simulink model "FourCellImplementation"  (R2020a)
settings: Solver=VariableStepAuto  StartTime=0.0  StopTime=10.0  RelTol=1e-3
libraries: powerlib x18
settings Model: Creator=HP  LastModifiedBy=HP

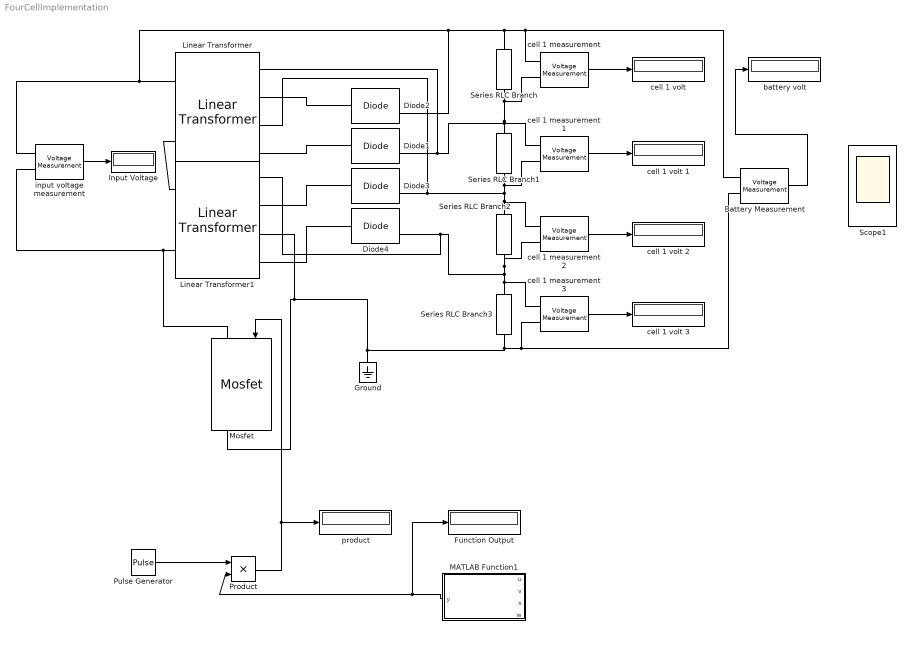
== system FourCellImplementation ==
  "Battery Measurement " : powerlib/Measurements/Voltage Measurement  PhasorSimulation=off  OutputType=Complex  PSBequivalent=0
  Diode{1..4} (4 alike) : powerlib/Power Electronics/Diode  Ron=0.001  Lon=0  Vf=0.8  IC=0  UseSnubber=0  Rs=500  Cs=250e-9  Measurements=on
  Function Output : Display
  Ground : powerlib/Elements/Ground  LConnTagsString=a
  Input Voltage : Display
  Linear Transformer : powerlib/Elements/Linear Transformer  UNITS=SI  NominalPower=[100 55000]  winding1=[10 0.02 45e-6]  winding2=[5 0.02 288e-6]  ThreeWindings=on  winding3=[5 0.02 288e-6]  RmLm=[1.0805e+06 2866]  Measurements=None  DataType=on
  Linear Transformer1 : powerlib/Elements/Linear Transformer  UNITS=SI  NominalPower=[100 55000]  winding1=[10 0.02 45e-6]  winding2=[5 0.02 288e-6]  ThreeWindings=on  winding3=[5 0.02 288e-6]  RmLm=[1.0805e+06 2866]  Measurements=None  DataType=on
  MATLAB Function1 : MATLAB Function  TreatAsAtomicUnit=on
  Mosfet : powerlib/Power Electronics/Mosfet  Ron=1.5  Lon=0  Rd=2  Vfd=0  IC=0  Rs=1500  Cs=288e-7  Measurements=on
  Product : Product
  Pulse Generator : DiscretePulseGenerator  PulseType=Time based  Period=10  PulseWidth=50
  Scope1 : Scope  NumInputPorts=5
  Series RLC Branch : powerlib/Elements/Series RLC Branch  LConnTagsString=__new0  RConnTagsString=__new0  BranchType=C  Resistance=1  Inductance=1e-3  SetiL0=off  InitialCurrent=0  Capacitance=5  Setx0=on  InitialVoltage=3  Measurements=None
  Series RLC Branch1 : powerlib/Elements/Series RLC Branch  LConnTagsString=__new0  RConnTagsString=__new0  BranchType=C  Resistance=1  Inductance=1e-3  SetiL0=off  InitialCurrent=0  Capacitance=5  Setx0=on  InitialVoltage=3.4  Measurements=None
  Series RLC Branch2 : powerlib/Elements/Series RLC Branch  LConnTagsString=__new0  RConnTagsString=__new0  BranchType=C  Resistance=1  Inductance=1e-3  SetiL0=off  InitialCurrent=0  Capacitance=5  Setx0=on  InitialVoltage=2.5  Measurements=None
  Series RLC Branch3 : powerlib/Elements/Series RLC Branch  LConnTagsString=__new0  RConnTagsString=__new0  BranchType=C  Resistance=1  Inductance=1e-3  SetiL0=off  InitialCurrent=0  Capacitance=5  Setx0=on  InitialVoltage=3.4  Measurements=None
  "battery volt " : Display
  cell 1 measurement {,1..3} (4 alike) : powerlib/Measurements/Voltage Measurement  PhasorSimulation=off  OutputType=Complex  PSBequivalent=0
  cell 1 volt {,1..3} (4 alike) : Display
  "input voltage measurement " : powerlib/Measurements/Voltage Measurement  PhasorSimulation=off  OutputType=Complex  PSBequivalent=0
  "product " : Display
  wires:
  "input voltage measurement "/1 -> Input Voltage/1
  Pulse Generator/1 -> Product/1
  Product/1 -> "product "/1, Mosfet/1
  MATLAB Function1/1(y) -> Function Output/1, Product/2
  "cell 1 measurement "/1 -> "cell 1 volt "/1
  cell 1 measurement 1/1 -> cell 1 volt 1/1
  cell 1 measurement 2/1 -> cell 1 volt 2/1
  cell 1 measurement 3/1 -> cell 1 volt 3/1
  "Battery Measurement "/1 -> "battery volt "/1
  connections:
  Linear Transformer/LConn2 -- Linear Transformer1/LConn1
  Series RLC Branch/LConn1 -- "Battery Measurement "/LConn1 -- "cell 1 measurement "/LConn1 -- Linear Transformer/LConn1 -- "input voltage measurement "/LConn1 -- Diode2/RConn1
  "input voltage measurement "/LConn2 -- Mosfet/LConn1 -- Linear Transformer1/LConn2
  Series RLC Branch3/LConn1 -- cell 1 measurement 3/LConn1 -- Linear Transformer1/RConn1 -- Diode4/RConn1 -- cell 1 measurement 2/LConn2 -- Series RLC Branch2/RConn1
  Series RLC Branch1/RConn1 -- cell 1 measurement 1/LConn2 -- Linear Transformer/RConn3 -- Diode3/RConn1 -- cell 1 measurement 2/LConn1 -- Series RLC Branch2/LConn1
  Series RLC Branch1/LConn1 -- cell 1 measurement 1/LConn1 -- Linear Transformer/RConn1 -- Diode1/RConn1 -- "cell 1 measurement "/LConn2 -- Series RLC Branch/RConn1
  Series RLC Branch3/RConn1 -- "Battery Measurement "/LConn2 -- cell 1 measurement 3/LConn2 -- Mosfet/RConn1 -- Linear Transformer1/RConn3 -- Ground/LConn1
  Linear Transformer/RConn2 -- Diode2/LConn1
  Linear Transformer/RConn4 -- Diode1/LConn1
  Linear Transformer1/RConn2 -- Diode3/LConn1
  Linear Transformer1/RConn4 -- Diode4/LConn1

== matlab function FourCellImplementation/MATLAB Function1 ==
  data: u input; y output; v input; x input; w input
function y = fcn(u,v,x,w)
if(u <= v && u >= v &&  v<= w && v>= w && v <= x && v >= x)
    y = 0;
else 
    y = 1;
end
